simulink model "test_com_SensorFusion_SF_D4"  (R2019b)
settings: Solver=FixedStepDiscrete  StartTime=0  StopTime=stop  FixedStep=0.001  RelTol=1e-3
undefined symbols (not defined in the file or in its folder): BxTM, ByTM, CxTM, CyTM, g, gamma_stat_front, gamma_stat_rear, gearbox_ratio, l_F, l_R, m_sprung, m_unsprung_quarter, mag_calib_front_center, mag_calib_front_compmatrix, mag_calib_rear_center, mag_calib_rear_compmatrix, should_be_in_theSensorFusion, switch_VelYcalculation_pSF, testStart_VelX_pSF, testVelY_pSF, tire_r_dyn, track_angle_front, track_width_front, track_width_rear, v2o_x, wheel_kinematics_breakpoints, wheel_kinematics_FL_data, wheel_kinematics_FR_data, wheelbase, x9DFrontX, x9DFrontY, x9DRearX, x9DRearY
libraries: SignalProcessingSensorFusionLib x30, simulink x6
(part 2 of 9)

== system test_com_SensorFusion_SF_D4/0213_PlausibiltyCheck1/9DRear_Plausibility ==
  In : Inport  OutDataTypeStr=Bus: control_9D
  Bus Creator : BusCreator  Inputs=16  OutDataTypeStr=Bus: control_9D
  Bus Selector : BusSelector  OutputSignals=AccX,AccX_Sq,AccY,AccY_Sq,AccZ,AccZ_Sq,RollRate,RollRate_Sq,PitchRate,PitchRate_Sq,YawRate,YawRate_Sq,MagX,MagY,MagZ,Temperature
  Plausibility_Test_AccX : SignalProcessingSensorFusionLib/Plausibility_AllTests  alpha=0.3  checkGradient=off  deviation=0  threshold=0  alpha2=0  increasingPercentage=0  signalBounds=1e-8  stepDelay=25  upperBound=50  lowerBound=-50  useAlternativeValue=off  useManualAlternativeValue=off  manualAlternativeValue=0
  Plausibility_Test_AccY : SignalProcessingSensorFusionLib/Plausibility_AllTests  alpha=0.3  checkGradient=off  deviation=0  threshold=0  alpha2=0  increasingPercentage=0  signalBounds=1e-8  stepDelay=25  upperBound=50  lowerBound=-50  useAlternativeValue=off  useManualAlternativeValue=off  manualAlternativeValue=0
  Plausibility_Test_AccZ : SignalProcessingSensorFusionLib/Plausibility_AllTests  alpha=0.3  checkGradient=off  deviation=0  threshold=0  alpha2=0  increasingPercentage=0  signalBounds=1e-8  stepDelay=25  upperBound=50  lowerBound=-50  useAlternativeValue=off  useManualAlternativeValue=off  manualAlternativeValue=0
  Plausibility_Test_PitchRate : SignalProcessingSensorFusionLib/Plausibility_AllTests  alpha=0.3  checkGradient=off  deviation=0  threshold=0  alpha2=0  increasingPercentage=0  signalBounds=1e-8  stepDelay=25  upperBound=1.5  lowerBound=-1.5  useAlternativeValue=off  useManualAlternativeValue=off  manualAlternativeValue=0
  Plausibility_Test_RollRate : SignalProcessingSensorFusionLib/Plausibility_AllTests  alpha=0.3  checkGradient=off  deviation=0  threshold=0  alpha2=0  increasingPercentage=0  signalBounds=1e-8  stepDelay=25  upperBound=1.5  lowerBound=-1.5  useAlternativeValue=off  useManualAlternativeValue=off  manualAlternativeValue=0
  Plausibility_Test_YawRate : SignalProcessingSensorFusionLib/Plausibility_AllTests  alpha=0.3  checkGradient=off  deviation=0  threshold=0  alpha2=0  increasingPercentage=0  signalBounds=1e-8  stepDelay=25  upperBound=4  lowerBound=-4  useAlternativeValue=off  useManualAlternativeValue=off  manualAlternativeValue=0
  Scope : Scope  NumInputPorts=2
  Out : Outport  VectorParamsAs1DForOutWhenUnconnected=off
  wires:
  Plausibility_Test_AccY/1 -> Bus Creator/2  "AccY"
  Bus Selector/2 -> Plausibility_Test_AccX/2  "<AccX_Sq>"
  Bus Selector/4 -> Plausibility_Test_AccY/2  "<AccY_Sq>"
  Bus Selector/3 -> Plausibility_Test_AccY/1  "<AccY>"
  In/1 -> Bus Selector/1
  Plausibility_Test_AccX/1 -> Bus Creator/1  "AccX"
  Bus Selector/1 -> Plausibility_Test_AccX/1  "<AccX>"
  Bus Selector/6 -> Plausibility_Test_AccZ/2  "<AccZ_Sq>"
  Plausibility_Test_AccZ/1 -> Scope/1, Bus Creator/3  "AccZ"
  Bus Selector/5 -> Plausibility_Test_AccZ/1  "<AccZ>"
  Bus Selector/8 -> Plausibility_Test_RollRate/2  "<RollRate_Sq>"
  Bus Selector/7 -> Plausibility_Test_RollRate/1  "<RollRate>"
  Plausibility_Test_RollRate/1 -> Bus Creator/4  "RollRate"
  Bus Creator/1 -> Out/1
  Bus Selector/10 -> Plausibility_Test_PitchRate/2  "<PitchRate_Sq>"
  Plausibility_Test_PitchRate/1 -> Bus Creator/5  "PitchRate"
  Bus Selector/12 -> Plausibility_Test_YawRate/2  "<YawRate_Sq>"
  Plausibility_Test_YawRate/1 -> Bus Creator/6  "YawRate"
  Bus Selector/9 -> Plausibility_Test_PitchRate/1  "<PitchRate>"
  Bus Selector/11 -> Plausibility_Test_YawRate/1  "<YawRate>"
  Bus Selector/13 -> Bus Creator/7  "<MagX>"
  Bus Selector/14 -> Bus Creator/8  "<MagY>"
  Bus Selector/15 -> Bus Creator/9  "<MagZ>"
  Bus Selector/16 -> Bus Creator/10  "<Temperature>"
  Plausibility_Test_PitchRate/2 -> Bus Creator/15  "PitchRate_Sq"
  Plausibility_Test_AccZ/2 -> Scope/2, Bus Creator/13  "AccZ_Sq"
  Plausibility_Test_YawRate/2 -> Bus Creator/16  "YawRate_Sq"
  Plausibility_Test_AccX/2 -> Bus Creator/11  "AccX_Sq"
  Plausibility_Test_RollRate/2 -> Bus Creator/14  "RollRate_Sq"
  Plausibility_Test_AccY/2 -> Bus Creator/12  "AccY_Sq"

== system test_com_SensorFusion_SF_D4/0213_PlausibiltyCheck1/DriverRequest_Plausibility ==
  In : Inport  OutDataTypeStr=Bus: control_DriverRequest
  Bus Creator : BusCreator  Inputs=11  OutDataTypeStr=Bus: control_DriverRequest
      settings: InheritFromInputs=off
  Bus Selector : BusSelector  OutputSignals=Pedal_BrakeMech_Value,Pedal_BrakeRecu_Value,SteeringwheelAngle,Pedal_Accel_Value,Pedal_TorqueValid_flag,Pedal_BrakeHard_flag,Pedal_BrakeMech_flag,SteeringValid_flag,Pedal_BrakeValid_flag,SteeringwheelAngle_Sq,Pedal_Accel_Value_Sq
  Data Type Conrsion{1..3,22} (4 alike) : DataTypeConversion  OutDataTypeStr=single
  Data Type Conrsion{4..7} (4 alike) : DataTypeConversion  OutDataTypeStr=uint8
  Plausibility_Test_SteeringwheelAngle : SignalProcessingSensorFusionLib/Plausibility_AllTests  alpha=0.3  checkGradient=off  deviation=0  threshold=0  alpha2=0  increasingPercentage=0  signalBounds=1e-10  stepDelay=40  upperBound=115  lowerBound=-115  useAlternativeValue=off  useManualAlternativeValue=off  manualAlternativeValue=0
  Plausibility_Test_SteeringwheelAngle3 : SignalProcessingSensorFusionLib/Plausibility_AllTests  alpha=0.3  checkGradient=off  deviation=0  threshold=0  alpha2=0  increasingPercentage=0  signalBounds=1e-10  stepDelay=40  upperBound=1  lowerBound=0  useAlternativeValue=off  useManualAlternativeValue=off  manualAlternativeValue=0
  Out : Outport  VectorParamsAs1DForOutWhenUnconnected=off
  wires:
  In/1 -> Bus Selector/1
  Bus Creator/1 -> Out/1
  Bus Selector/1 -> Data Type Conrsion22/1  "<Pedal_BrakeMech_Value>"
  Bus Selector/2 -> Data Type Conrsion1/1  "<Pedal_BrakeRecu_Value>"
  Bus Selector/3 -> Plausibility_Test_SteeringwheelAngle/1  "<SteeringwheelAngle>"
  Plausibility_Test_SteeringwheelAngle/1 -> Data Type Conrsion2/1  "SteeringwheelAngle"
  Bus Selector/4 -> Plausibility_Test_SteeringwheelAngle3/1  "<Pedal_Accel_Value>"
  Bus Selector/5 -> Bus Creator/5  "<Pedal_TorqueValid_flag>"
  Bus Selector/6 -> Bus Creator/6  "<Pedal_BrakeHard_flag>"
  Bus Selector/7 -> Bus Creator/7  "<Pedal_BrakeMech_flag>"
  Bus Selector/8 -> Bus Creator/8  "<SteeringValid_flag>"
  Bus Selector/9 -> Bus Creator/9  "<Pedal_BrakeValid_flag>"
  Plausibility_Test_SteeringwheelAngle/2 -> Data Type Conrsion4/1  "SteeringwheelAngle_Sq"
  Plausibility_Test_SteeringwheelAngle3/1 -> Data Type Conrsion3/1
  Bus Selector/10 -> Data Type Conrsion6/1  "<SteeringwheelAngle_Sq>"
  Data Type Conrsion22/1 -> Bus Creator/1
  Data Type Conrsion1/1 -> Bus Creator/2
  Data Type Conrsion2/1 -> Bus Creator/3
  Data Type Conrsion3/1 -> Bus Creator/4
  Data Type Conrsion4/1 -> Bus Creator/10
  Bus Selector/11 -> Data Type Conrsion7/1  "<Pedal_Accel_Value_Sq>"
  Plausibility_Test_SteeringwheelAngle3/2 -> Data Type Conrsion5/1
  Data Type Conrsion5/1 -> Bus Creator/11
  Data Type Conrsion6/1 -> Plausibility_Test_SteeringwheelAngle/2
  Data Type Conrsion7/1 -> Plausibility_Test_SteeringwheelAngle3/2

== system test_com_SensorFusion_SF_D4/0213_PlausibiltyCheck1/Suspension_Plausibility ==
  In : Inport  OutDataTypeStr=Bus: control_Suspension
  Bus Creator : BusCreator  Inputs=8  OutDataTypeStr=Bus: control_Suspension
  Bus Selector : BusSelector  OutputSignals=RockerAngle_FL,RockerAngle_FL_Sq,RockerAngle_FR,RockerAngle_FR_Sq,RockerAngle_RL,RockerAngle_RL_Sq,RockerAngle_RR,RockerAngle_RR_Sq
  Data Type Conrsion{1..3,22} (4 alike) : DataTypeConversion  OutDataTypeStr=single
  Plausibility_Test_RockerAngle_FL : SignalProcessingSensorFusionLib/Plausibility_AllTests  alpha=0  checkGradient=off  deviation=0  threshold=0  alpha2=0  increasingPercentage=0  signalBounds=1e-10  stepDelay=38  upperBound=30  lowerBound=-30  useAlternativeValue=off  useManualAlternativeValue=off  manualAlternativeValue=0
  Plausibility_Test_RockerAngle_FR : SignalProcessingSensorFusionLib/Plausibility_AllTests  alpha=0  checkGradient=off  deviation=0  threshold=0  alpha2=0  increasingPercentage=0  signalBounds=1e-10  stepDelay=38  upperBound=30  lowerBound=-30  useAlternativeValue=off  useManualAlternativeValue=off  manualAlternativeValue=0
  Plausibility_Test_RockerAngle_RL : SignalProcessingSensorFusionLib/Plausibility_AllTests  alpha=0  checkGradient=off  deviation=0  threshold=0  alpha2=0  increasingPercentage=0  signalBounds=1e-10  stepDelay=38  upperBound=30  lowerBound=-30  useAlternativeValue=off  useManualAlternativeValue=off  manualAlternativeValue=0
  Plausibility_Test_RockerAngle_RR : SignalProcessingSensorFusionLib/Plausibility_AllTests  alpha=0  checkGradient=off  deviation=0  threshold=0  alpha2=0  increasingPercentage=0  signalBounds=1e-10  stepDelay=38  upperBound=30  lowerBound=-30  useAlternativeValue=off  useManualAlternativeValue=off  manualAlternativeValue=0
  Out : Outport  VectorParamsAs1DForOutWhenUnconnected=off
  wires:
  Plausibility_Test_RockerAngle_FL/2 -> Bus Creator/5  "RockerAngle_FL_Sq"
  Plausibility_Test_RockerAngle_FR/2 -> Bus Creator/6  "RockerAngle_FR_Sq"
  Plausibility_Test_RockerAngle_RL/2 -> Bus Creator/7  "RockerAngle_RL_Sq"
  Bus Selector/6 -> Plausibility_Test_RockerAngle_RL/2  "<RockerAngle_RL_Sq>"
  Bus Selector/5 -> Plausibility_Test_RockerAngle_RL/1  "<RockerAngle_RL>"
  Bus Selector/4 -> Plausibility_Test_RockerAngle_FR/2  "<RockerAngle_FR_Sq>"
  Bus Selector/3 -> Plausibility_Test_RockerAngle_FR/1  "<RockerAngle_FR>"
  Bus Selector/2 -> Plausibility_Test_RockerAngle_FL/2  "<RockerAngle_FL_Sq>"
  Bus Selector/1 -> Plausibility_Test_RockerAngle_FL/1  "<RockerAngle_FL>"
  Bus Creator/1 -> Out/1
  Plausibility_Test_RockerAngle_RL/1 -> Data Type Conrsion2/1
  Plausibility_Test_RockerAngle_FL/1 -> Data Type Conrsion22/1
  In/1 -> Bus Selector/1
  Plausibility_Test_RockerAngle_FR/1 -> Data Type Conrsion1/1
  Bus Selector/7 -> Plausibility_Test_RockerAngle_RR/1  "<RockerAngle_RR>"
  Plausibility_Test_RockerAngle_RR/2 -> Bus Creator/8  "RockerAngle_RR_Sq"
  Plausibility_Test_RockerAngle_RR/1 -> Data Type Conrsion3/1
  Bus Selector/8 -> Plausibility_Test_RockerAngle_RR/2  "<RockerAngle_RR_Sq>"
  Data Type Conrsion22/1 -> Bus Creator/1  "RockerAngle_FL"
  Data Type Conrsion1/1 -> Bus Creator/2  "RockerAngle_FR"
  Data Type Conrsion2/1 -> Bus Creator/3  "RockerAngle_RL"
  Data Type Conrsion3/1 -> Bus Creator/4  "RockerAngle_RR"

== system test_com_SensorFusion_SF_D4/0213_PlausibiltyCheck1/Suspension_Plausibility1 ==
  In : Inport  OutDataTypeStr=Bus: control_Electric
  Bus Creator : BusCreator  Inputs=12  OutDataTypeStr=Bus: control_Electric
  Bus Selector : BusSelector  OutputSignals=BatSOC,BatVoltage,BatPower,BatCurrent,AvgCellVoltage,MaxCellVoltage,MinCellVoltage,IVTEnergy,MinCellTemp,IVT_VoltageCurrent_Sq,IVT_Energy_Sq,HVM_BMS_Sq
  Data Type Conrsion22 : DataTypeConversion  OutDataTypeStr=single
  Plausibility_Test_RockerAngle_RL : SignalProcessingSensorFusionLib/Plausibility_AllTests  alpha=0  checkGradient=off  deviation=0  threshold=0  alpha2=0  increasingPercentage=0  signalBounds=1e-10  stepDelay=40  upperBound=120000  lowerBound=-120000  useAlternativeValue=off  useManualAlternativeValue=off  manualAlternativeValue=0
  Out : Outport  VectorParamsAs1DForOutWhenUnconnected=off
  wires:
  Bus Selector/8 -> Plausibility_Test_RockerAngle_RL/1  "<IVTEnergy>"
  Bus Selector/7 -> Bus Creator/7  "<MinCellVoltage>"
  In/1 -> Bus Selector/1
  Bus Creator/1 -> Out/1
  Bus Selector/1 -> Bus Creator/1  "<BatSOC>"
  Bus Selector/2 -> Bus Creator/2  "<BatVoltage>"
  Bus Selector/3 -> Bus Creator/3  "<BatPower>"
  Bus Selector/4 -> Bus Creator/4  "<BatCurrent>"
  Bus Selector/5 -> Bus Creator/5  "<AvgCellVoltage>"
  Bus Selector/6 -> Bus Creator/6  "<MaxCellVoltage>"
  Bus Selector/9 -> Bus Creator/9  "<MinCellTemp>"
  Bus Selector/10 -> Bus Creator/10  "<IVT_VoltageCurrent_Sq>"
  Bus Selector/11 -> Plausibility_Test_RockerAngle_RL/2  "<IVT_Energy_Sq>"
  Bus Selector/12 -> Bus Creator/12  "<HVM_BMS_Sq>"
  Plausibility_Test_RockerAngle_RL/2 -> Bus Creator/11  "AccZ_Sq"
  Plausibility_Test_RockerAngle_RL/1 -> Data Type Conrsion22/1  "VelZ"
  Data Type Conrsion22/1 -> Bus Creator/8

== system test_com_SensorFusion_SF_D4/0213_PlausibiltyCheck1/motorSpeed_Plausibility ==
  In : Inport
  Constant{,1..3} (4 alike) : Constant  Value=uint8(0)
  Data Type Conrsion22 : DataTypeConversion  OutDataTypeStr=single
  Demux : Demux
  Mux : Mux
  Mux1 : Mux
  Plausibility_Test_AccX : SignalProcessingSensorFusionLib/Plausibility_AllTests  alpha=0  checkGradient=off  deviation=0  threshold=0  alpha2=0  increasingPercentage=0  signalBounds=1e-10  stepDelay=40  upperBound=20000  lowerBound=-10000  useAlternativeValue=off  useManualAlternativeValue=off  manualAlternativeValue=0
  Plausibility_Test_AccY : SignalProcessingSensorFusionLib/Plausibility_AllTests  alpha=0  checkGradient=off  deviation=0  threshold=0  alpha2=0  increasingPercentage=0  signalBounds=1e-10  stepDelay=40  upperBound=20000  lowerBound=-10000  useAlternativeValue=off  useManualAlternativeValue=off  manualAlternativeValue=0
  Plausibility_Test_AccZ : SignalProcessingSensorFusionLib/Plausibility_AllTests  alpha=0  checkGradient=off  deviation=0  threshold=0  alpha2=0  increasingPercentage=0  signalBounds=1e-10  stepDelay=40  upperBound=20000  lowerBound=-10000  useAlternativeValue=off  useManualAlternativeValue=off  manualAlternativeValue=0
  Plausibility_Test_AccZ1 : SignalProcessingSensorFusionLib/Plausibility_AllTests  alpha=0  checkGradient=off  deviation=0  threshold=0  alpha2=0  increasingPercentage=0  signalBounds=1e-10  stepDelay=40  upperBound=20000  lowerBound=-10000  useAlternativeValue=off  useManualAlternativeValue=off  manualAlternativeValue=0
  WheelSpeed : Outport  VectorParamsAs1DForOutWhenUnconnected=off
  WheelSpeed_Sq : Outport  Port=2  VectorParamsAs1DForOutWhenUnconnected=off
  wires:
  Plausibility_Test_AccX/2 -> Mux1/1  "AccX_Sq"
  Plausibility_Test_AccZ1/2 -> Mux1/4
  Mux1/1 -> WheelSpeed_Sq/1
  Mux/1 -> Data Type Conrsion22/1
  Plausibility_Test_AccZ1/1 -> Mux/4
  Constant3/1 -> Plausibility_Test_AccZ1/2
  Constant2/1 -> Plausibility_Test_AccZ/2
  Constant1/1 -> Plausibility_Test_AccY/2
  Constant/1 -> Plausibility_Test_AccX/2
  Demux/4 -> Plausibility_Test_AccZ1/1
  Plausibility_Test_AccY/2 -> Mux1/2  "AccY_Sq"
  Plausibility_Test_AccZ/2 -> Mux1/3  "AccZ_Sq"
  Demux/3 -> Plausibility_Test_AccZ/1
  Demux/2 -> Plausibility_Test_AccY/1
  Demux/1 -> Plausibility_Test_AccX/1
  Plausibility_Test_AccZ/1 -> Mux/3  "VelZ"
  Plausibility_Test_AccX/1 -> Mux/1  "VelX"
  In/1 -> Demux/1  "wheelSpeed"
  Plausibility_Test_AccY/1 -> Mux/2  "VelY"
  Data Type Conrsion22/1 -> WheelSpeed/1

== system test_com_SensorFusion_SF_D4/0213_PlausibiltyCheck1/v2oVelocity_Plausibility ==
  In : Inport  OutDataTypeStr=Bus: control_Velocity
  Bus Creator : BusCreator  Inputs=7  OutDataTypeStr=Bus: control_Velocity
  Bus Creator1 : BusCreator  Inputs=2
  Bus Creator2 : BusCreator  Inputs=2
  Bus Selector : BusSelector  OutputSignals=SlipAngle,SlipAngle_Sq,VelY,VelY_Sq,VelX,VelX_Sq,valueIsNew
  Bus Selector1 : BusSelector  OutputSignals=VelY,VelX,VelY_Sq,VelX_Sq
  Data Type Conrsion1 : DataTypeConversion  OutDataTypeStr=single
  Data Type Conrsion2 : DataTypeConversion  OutDataTypeStr=single
  Data Type Conrsion22 : DataTypeConversion  OutDataTypeStr=single
  Plausibility_Test_SlipAngle : SignalProcessingSensorFusionLib/Plausibility_AllTests  alpha=0  checkGradient=off  deviation=0  threshold=0  alpha2=0  increasingPercentage=0  signalBounds=1e-8  stepDelay=35  upperBound=90  lowerBound=-90  useAlternativeValue=off  useManualAlternativeValue=off  manualAlternativeValue=0
  Plausibility_Test_VelX : SignalProcessingSensorFusionLib/Plausibility_AllTests  alpha=0  checkGradient=off  deviation=0  threshold=0  alpha2=0  increasingPercentage=0  signalBounds=1e-8  stepDelay=35  upperBound=35  lowerBound=-3  useAlternativeValue=off  useManualAlternativeValue=off  manualAlternativeValue=0
  Plausibility_Test_VelY : SignalProcessingSensorFusionLib/Plausibility_AllTests  alpha=0  checkGradient=off  deviation=0  threshold=0  alpha2=0  increasingPercentage=0  signalBounds=1e-8  stepDelay=35  upperBound=50  lowerBound=-50  useAlternativeValue=off  useManualAlternativeValue=off  manualAlternativeValue=0
  Scope : Scope  NumInputPorts=2
  Out : Outport  VectorParamsAs1DForOutWhenUnconnected=off
  wires:
  Plausibility_Test_VelY/1 -> Data Type Conrsion22/1  "VelY"
  In/1 -> Bus Selector/1
  Plausibility_Test_SlipAngle/1 -> Data Type Conrsion1/1  "SlipAngle"
  Plausibility_Test_VelX/1 -> Data Type Conrsion2/1  "VelX"
  Bus Creator/1 -> Bus Selector1/1, Out/1
  Bus Selector/1 -> Plausibility_Test_SlipAngle/1  "<SlipAngle>"
  Bus Selector/2 -> Plausibility_Test_SlipAngle/2  "<SlipAngle_Sq>"
  Bus Selector/3 -> Plausibility_Test_VelY/1  "<VelY>"
  Bus Selector/4 -> Plausibility_Test_VelY/2  "<VelY_Sq>"
  Bus Selector/5 -> Plausibility_Test_VelX/1  "<VelX>"
  Bus Selector/6 -> Plausibility_Test_VelX/2  "<VelX_Sq>"
  Bus Selector/7 -> Bus Creator/7  "<valueIsNew>"
  Plausibility_Test_VelX/2 -> Bus Creator/6  "VelX_Sq"
  Plausibility_Test_VelY/2 -> Bus Creator/5  "VelY_Sq"
  Plausibility_Test_SlipAngle/2 -> Bus Creator/4  "SlipAngle_Sq"
  Data Type Conrsion22/1 -> Bus Creator/2  "VelY"
  Data Type Conrsion1/1 -> Bus Creator/1  "SlipAngle"
  Data Type Conrsion2/1 -> Bus Creator/3  "VelX"
  Bus Selector1/1 -> Bus Creator1/1  "<VelY>"
  Bus Selector1/2 -> Bus Creator1/2  "<VelX>"
  Bus Selector1/3 -> Bus Creator2/1  "<VelY_Sq>"
  Bus Selector1/4 -> Bus Creator2/2  "<VelX_Sq>"
  Bus Creator2/1 -> Scope/2
  Bus Creator1/1 -> Scope/1

== system test_com_SensorFusion_SF_D4/0213_PlausibiltyCheck1/wheelSpeed_Plausibility ==
  In : Inport
  Constant{,1..3} (4 alike) : Constant  Value=uint8(0)
  Data Type Conrsion{1..3,22} (4 alike) : DataTypeConversion  OutDataTypeStr=single
  Demux : Demux
  Mux : Mux
  Mux1 : Mux
  Plausibility_Test_WheelSpeed_FL : SignalProcessingSensorFusionLib/Plausibility_AllTests  alpha=0  checkGradient=off  deviation=0  threshold=0  alpha2=0  increasingPercentage=0  signalBounds=1e-12  stepDelay=40  upperBound=100  lowerBound=-10  useAlternativeValue=off  useManualAlternativeValue=off  manualAlternativeValue=0
  Plausibility_Test_WheelSpeed_FR : SignalProcessingSensorFusionLib/Plausibility_AllTests  alpha=0  checkGradient=off  deviation=0  threshold=0  alpha2=0  increasingPercentage=0  signalBounds=1e-12  stepDelay=40  upperBound=100  lowerBound=-10  useAlternativeValue=off  useManualAlternativeValue=off  manualAlternativeValue=0
  Plausibility_Test_WheelSpeed_RL : SignalProcessingSensorFusionLib/Plausibility_AllTests  alpha=0  checkGradient=off  deviation=0  threshold=0  alpha2=0  increasingPercentage=0  signalBounds=1e-12  stepDelay=40  upperBound=100  lowerBound=-10  useAlternativeValue=off  useManualAlternativeValue=off  manualAlternativeValue=0
  Plausibility_Test_WheelSpeed_RR : SignalProcessingSensorFusionLib/Plausibility_AllTests  alpha=0  checkGradient=off  deviation=0  threshold=0  alpha2=0  increasingPercentage=0  signalBounds=1e-12  stepDelay=40  upperBound=100  lowerBound=-10  useAlternativeValue=off  useManualAlternativeValue=off  manualAlternativeValue=0
  WheelSpeed : Outport  VectorParamsAs1DForOutWhenUnconnected=off
  WheelSpeed_Sq : Outport  Port=2  VectorParamsAs1DForOutWhenUnconnected=off
  wires:
  Plausibility_Test_WheelSpeed_FR/1 -> Data Type Conrsion1/1  "VelY"
  In/1 -> Demux/1  "wheelSpeed"
  Plausibility_Test_WheelSpeed_FL/1 -> Data Type Conrsion22/1  "VelX"
  Plausibility_Test_WheelSpeed_RL/1 -> Data Type Conrsion2/1  "VelZ"
  Demux/1 -> Plausibility_Test_WheelSpeed_FL/1
  Demux/2 -> Plausibility_Test_WheelSpeed_FR/1
  Demux/3 -> Plausibility_Test_WheelSpeed_RL/1
  Plausibility_Test_WheelSpeed_RL/2 -> Mux1/3  "AccZ_Sq"
  Plausibility_Test_WheelSpeed_FR/2 -> Mux1/2  "AccY_Sq"
  Demux/4 -> Plausibility_Test_WheelSpeed_RR/1
  Constant/1 -> Plausibility_Test_WheelSpeed_FL/2
  Constant1/1 -> Plausibility_Test_WheelSpeed_FR/2
  Constant2/1 -> Plausibility_Test_WheelSpeed_RL/2
  Constant3/1 -> Plausibility_Test_WheelSpeed_RR/2
  Plausibility_Test_WheelSpeed_RR/1 -> Data Type Conrsion3/1
  Mux/1 -> WheelSpeed/1
  Mux1/1 -> WheelSpeed_Sq/1
  Plausibility_Test_WheelSpeed_RR/2 -> Mux1/4
  Plausibility_Test_WheelSpeed_FL/2 -> Mux1/1  "AccX_Sq"
  Data Type Conrsion22/1 -> Mux/1
  Data Type Conrsion1/1 -> Mux/2
  Data Type Conrsion2/1 -> Mux/3
  Data Type Conrsion3/1 -> Mux/4

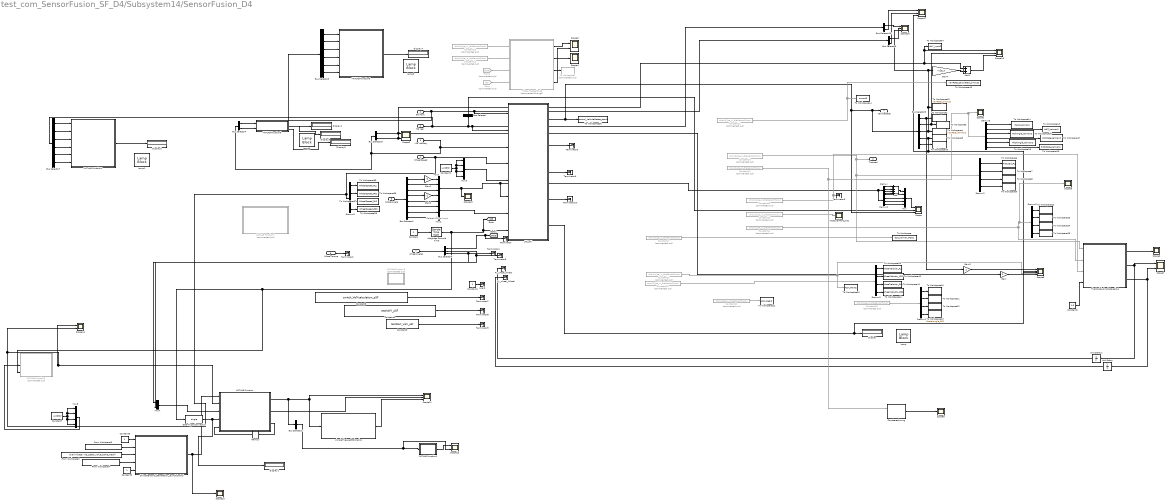
== system test_com_SensorFusion_SF_D4/Subsystem14/SensorFusion_D4 ==
  note: Deleted Driver Input
  9D front : Inport
  9D rear : Inport  Port=2
  v2o velocity : Inport  Port=3
  WheelSpeed : Inport  Port=4
  RockerAngle : Inport  Port=5
  WheelTorque : Inport  Port=6
  WheelAngle1 : Inport  Port=7
  Add : Sum  Inputs=++++
  Add1 : Sum
  Bus Selector : BusSelector  OutputSignals=AccX,AccY,AccZ,RollRate,PitchRate,YawRate  OutputAsBus=on
  Bus Selector1 : BusSelector  OutputSignals=RockerAngle_FL,RockerAngle_FR,RockerAngle_RL,RockerAngle_RR,RockerAngle_FL_Sq,RockerAngle_FR_Sq,RockerAngle_RL_Sq,RockerAngle_RR_Sq
  Bus Selector10 : BusSelector  OutputSignals=YawRate,AccX
  Bus Selector2 : BusSelector  OutputSignals=AccX
  Bus Selector3 : BusSelector  OutputSignals=VelX,VelY
  Bus Selector4 : BusSelector  OutputSignals=VelX_Sq,VelY_Sq
  Bus Selector5 : BusSelector  OutputSignals=VelX,VelY,YawRate,AccX,AccY
  Bus Selector6 : BusSelector  OutputSignals=WheelAngle_AVG,WheelAngle_FL,WheelAngle_FR
  Bus Selector7 : BusSelector  OutputSignals=AccX_Sq,AccY_Sq,AccZ_Sq,YawRate_Sq,PitchRate_Sq,RollRate_Sq
  Bus Selector8 : BusSelector  OutputSignals=AccX_Sq,AccY_Sq,AccZ_Sq,YawRate_Sq,PitchRate_Sq,RollRate_Sq
  Bus Selector9 : BusSelector  OutputSignals=YawRate,AccX
  Constant{,4..6} (4 alike) : Constant
  Constant1 : Constant  Value=uint8(0)
  Constant{10..22} (13 alike) : Constant  Commented=on  Value=should_be_in_theSensorFusion
  Constant2 : Constant  Value=1.6
  Constant3 : Constant  Value=testVelY_pSF
  Constant7 : Constant  Value=uint8(0)
  Constant8 : Constant  Value=switch_VelYcalculation_pSF
  Constant9 : Constant  Value=testStart_VelX_pSF
  Data Type Conversion : DataTypeConversion  OutDataTypeStr=single
  Demux{,1..2,4..5,8..9} (7 alike) : Demux
  Demux3 : Demux  Outputs=6
  Display{,1..6} (7 alike) : Display
  DriverDemand_Generation_LaunchControl : Subsystem
  From : From  Commented=on  GotoTag=dt
  From Workspace2 : FromWorkspace  VariableName=evalin('base','VD_pedal_value_brake_mech')  SampleTime=0
  From Workspace3 : FromWorkspace  VariableName=evalin('base','VD_pedal_value_brake_rec')  SampleTime=0
  From Workspace4 : FromWorkspace  VariableName=evalin('base','VD_pedal_value_torque')  SampleTime=0
  From1 : From  Commented=on  GotoTag=delta
  Fx_wheel_Wheel : Terminator
  Fy_wheel_Wheel : Terminator
  Gain : Gain  OutDataTypeStr=single
  Gain1 : Gain  Gain=-1
  Gain2 : Gain  Gain=-1
  Gain3 : Gain  OutDataTypeStr=single
  Gain4 : Gain  Gain=-v2o_x
  Lamp{,1..3} (4 alike) : LampBlock
  MATLAB Function : MATLAB Function  TreatAsAtomicUnit=on
  MATLAB Function1 : MATLAB Function  TreatAsAtomicUnit=on
  MATLAB Function2 : MATLAB Function  Commented=on  TreatAsAtomicUnit=on
  MATLAB Function3 : MATLAB Function  Commented=on  TreatAsAtomicUnit=on
  MATLAB Function4 : MATLAB Function  TreatAsAtomicUnit=on
  MATLAB Function5 : MATLAB Function  TreatAsAtomicUnit=on
  MATLAB Function6 : MATLAB Function  TreatAsAtomicUnit=on
  MATLAB Function7 : MATLAB Function  Commented=on  TreatAsAtomicUnit=on
  Memory : Memory
  Mux : Mux  Inputs=5
  Mux{1..3,5} (4 alike) : Mux
  Mux4 : Mux  Inputs=2
  SF_LaKl : MATLAB Function  TreatAsAtomicUnit=on
  Scope{,11,15..17} (5 alike) : Scope  NumInputPorts=3
  Scope{1..2,4,6,9..10,13} (7 alike) : Scope
  Scope{3,5,7,12,14} (5 alike) : Scope  NumInputPorts=2
  Scope8 : Scope  NumInputPorts=5
  SiDes Testgelände : MATLAB Function  Commented=through  TreatAsAtomicUnit=on
  Sturzberechnung : Subsystem
  Terminator{,1..10} (11 alike) : Terminator
  TireModel_simplePacejka1 : MATLAB Function  TreatAsAtomicUnit=on
  To Workspace : ToWorkspace  VariableName=e10_kalman_POS2  SaveFormat=Timeseries  SampleTime=-1
  To Workspace1 : ToWorkspace  Commented=on  VariableName=e10_easy_POS  SaveFormat=Timeseries  SampleTime=-1
  To Workspace10 : ToWorkspace  VariableName=RockerAngle_FL2  SaveFormat=Timeseries  SampleTime=-1
  To Workspace11 : ToWorkspace  VariableName=RockerAngle_FR2  SaveFormat=Timeseries  SampleTime=-1
  To Workspace12 : ToWorkspace  VariableName=RockerAngle_RL2  SaveFormat=Timeseries  SampleTime=-1
  To Workspace13 : ToWorkspace  VariableName=RockerAngle_RR2  SaveFormat=Timeseries  SampleTime=-1
  To Workspace14 : ToWorkspace  VariableName=PosZ_kalman2  SaveFormat=Timeseries  SampleTime=-1
  To Workspace15 : ToWorkspace  VariableName=VelZ_kalman2  SaveFormat=Timeseries  SampleTime=-1
  To Workspace16 : ToWorkspace  VariableName=RollAngle_kalman2  SaveFormat=Timeseries  SampleTime=-1
  To Workspace17 : ToWorkspace  VariableName=RollRate_kalman2  SaveFormat=Timeseries  SampleTime=-1
  To Workspace18 : ToWorkspace  VariableName=PitchAngle_kalman2  SaveFormat=Timeseries  SampleTime=-1
  To Workspace19 : ToWorkspace  VariableName=PitchRate_kalman2  SaveFormat=Timeseries  SampleTime=-1
  To Workspace2 : ToWorkspace  VariableName=VelX_kalman2  SaveFormat=Timeseries  SampleTime=-1
  To Workspace20 : ToWorkspace  VariableName=AccX_Front2  SaveFormat=Timeseries  SampleTime=-1
  To Workspace21 : ToWorkspace  VariableName=AccX_Rear2  SaveFormat=Timeseries  SampleTime=-1
  To Workspace22 : ToWorkspace  VariableName=TireSlipLong_FL2  SaveFormat=Timeseries  SampleTime=-1
  To Workspace23 : ToWorkspace  VariableName=TireSlipLong_FR2  SaveFormat=Timeseries  SampleTime=-1
  To Workspace24 : ToWorkspace  VariableName=TireSlipLong_RL2  SaveFormat=Timeseries  SampleTime=-1
  To Workspace25 : ToWorkspace  VariableName=TireSlipLong_RR2  SaveFormat=Timeseries  SampleTime=-1
  To Workspace26 : ToWorkspace  VariableName=control_VehicleStates_result  SaveFormat=Timeseries  SampleTime=-1
  To Workspace3 : ToWorkspace  VariableName=VelY_kalman2  SaveFormat=Timeseries  SampleTime=-1
  To Workspace34 : ToWorkspace  VariableName=VelY_input2  SaveFormat=Timeseries  SampleTime=-1
  To Workspace35 : ToWorkspace  VariableName=WheelSpeed_FL2  SaveFormat=Timeseries  SampleTime=-1
  To Workspace36 : ToWorkspace  VariableName=WheelSpeed_FR2  SaveFormat=Timeseries  SampleTime=-1
  To Workspace37 : ToWorkspace  VariableName=WheelSpeed_RL2  SaveFormat=Timeseries  SampleTime=-1
  To Workspace38 : ToWorkspace  VariableName=WheelSpeed_RR2  SaveFormat=Timeseries  SampleTime=-1
  To Workspace39 : ToWorkspace  VariableName=WheelVelocity_FL2  SaveFormat=Timeseries  SampleTime=-1
  To Workspace4 : ToWorkspace  VariableName=YawRate_kalman2  SaveFormat=Timeseries  SampleTime=-1
  To Workspace40 : ToWorkspace  VariableName=WheelVelocity_FR2  SaveFormat=Timeseries  SampleTime=-1
  To Workspace41 : ToWorkspace  VariableName=WheelVelocity_RL2  SaveFormat=Timeseries  SampleTime=-1
  To Workspace42 : ToWorkspace  VariableName=WheelVelocity_RR2  SaveFormat=Timeseries  SampleTime=-1
  To Workspace43 : ToWorkspace  VariableName=AccY_kalman2  SaveFormat=Timeseries  SampleTime=-1
  To Workspace44 : ToWorkspace  VariableName=simout2  SaveFormat=Timeseries  SampleTime=-1
  To Workspace45 : ToWorkspace  VariableName=YawRate_simout2  SaveFormat=Timeseries  SampleTime=-1
  To Workspace46 : ToWorkspace  VariableName=YawRate_Calculated_simout2  SaveFormat=Timeseries  SampleTime=-1
  To Workspace5 : ToWorkspace  VariableName=AccX_kalman2  SaveFormat=Timeseries  SampleTime=-1
  To Workspace6 : ToWorkspace  VariableName=TireLoad_FL2  SaveFormat=Timeseries  SampleTime=-1
  To Workspace7 : ToWorkspace  VariableName=TireLoad_FR2  SaveFormat=Timeseries  SampleTime=-1
  To Workspace8 : ToWorkspace  VariableName=TireLoad_RL2  SaveFormat=Timeseries  SampleTime=-1
  To Workspace9 : ToWorkspace  VariableName=TireLoad_RR2  SaveFormat=Timeseries  SampleTime=-1
  Unit Delay : UnitDelay  SampleTime=-1  HasFrameUpgradeWarning=on
  Unit Delay1 : UnitDelay  SampleTime=-1  HasFrameUpgradeWarning=on
  Weighted Sample Time : SampleTimeMath  TsampMathOp=Ts Only
  c_reib : Terminator
  measurement_bias : Scope
  simpleTireLoadEstimation : Subsystem
  VehicleState : Outport  VectorParamsAs1DForOutWhenUnconnected=off
  TireLoad : Outport  Port=2  VectorParamsAs1DForOutWhenUnconnected=off
  wires:
  Mux/1 -> Scope/1
  Demux1/4 -> Mux/5
  Demux1/3 -> Mux/4
  Demux1/2 -> Mux/3
  Demux1/1 -> Mux/2
  Add/1 -> Mux/1
  Demux/1 -> Add/1
  Demux/2 -> Add/2
  Demux/3 -> Add/3
  Demux/4 -> Add/4
  Bus Selector/1 -> Scope/2
  Gain2/1 -> Mux1/4
  Weighted Sample Time/1 -> MATLAB Function2/3(dt), Data Type Conversion/1, [dt], SF_LaKl/8(dt)
  Mux2/1 -> SF_LaKl/7(RockerAngle_Sq)
  Mux1/1 -> Scope10/1, Demux/1, Demux1/1, SF_LaKl/6(RockerAngle)
  Mux3/1 -> SF_LaKl/5(WheelSpeeds_Sq)
  Gain1/1 -> Mux1/1
  v2o velocity/1 -> SF_LaKl/3(v2o), Bus Selector4/1, Bus Selector3/1
  9D rear/1 -> Bus Selector7/1, Bus Selector10/1, SF_LaKl/2(x9DRear), Bus Selector/1
  Bus Selector1/5 -> Mux2/1  "<RockerAngle_FL_Sq>"
  Constant/1 -> Weighted Sample Time/1
  Constant1/1 -> Mux3/2, Mux3/1, Mux3/3, Mux3/4
  Constant10/1 -> TireModel_simplePacejka1/1(TireLoad), Demux2/1, TireLoad/1  "TireLoad"
  Bus Selector1/7 -> Mux2/3  "<RockerAngle_RL_Sq>"
  Bus Selector1/8 -> Mux2/4  "<RockerAngle_RR_Sq>"
  Bus Selector1/3 -> Mux1/3  "<RockerAngle_RL>"
  Bus Selector1/4 -> Gain2/1  "<RockerAngle_RR>"
  WheelTorque/1 -> Terminator1/1
  RockerAngle/1 -> Bus Selector1/1  "rockerAngle"
  Bus Selector1/1 -> Gain1/1  "<RockerAngle_FL>"
  Bus Selector1/2 -> Mux1/2  "<RockerAngle_FR>"
  Constant13/1 -> SiDes Testgelände/2(x)
  SF_LaKl/1(VehicleState) -> To Workspace26/1, Scope/3, Bus Selector5/1, VehicleState/1  "VehicleState"
  Bus Selector1/6 -> Mux2/2  "<RockerAngle_FR_Sq>"
  Constant17/1 -> To Workspace/1
  Constant16/1 -> measurement_bias/1
  Constant19/1 -> SiDes Testgelände/1(measurements_nb)
  SiDes Testgelände/3(easyPos_out) -> To Workspace1/1
  SiDes Testgelände/1(easyYawRate_out) -> Scope3/1
  SiDes Testgelände/2(easyYawAngle_out) -> Scope4/1
  From/1 -> SiDes Testgelände/4(dt)
  From1/1 -> SiDes Testgelände/3(delta)
  SiDes Testgelände/4(YawRateBySteer) -> Scope3/2
  Bus Selector3/1 -> Gain/1, Scope5/1  "<VelX>"
  Bus Selector3/2 -> Add1/1, Scope15/1, To Workspace34/1, Scope5/2  "<VelY>"
  Bus Selector6/2 -> Terminator5/1, Mux4/1  "<WheelAngle_FL>"
  Bus Selector6/3 -> Terminator4/1, Mux4/2  "<WheelAngle_FR>"
  WheelAngle1/1 -> Bus Selector6/1
  Bus Selector6/1 -> Terminator/1, [delta]  "<WheelAngle_AVG>"
  9D front/1 -> Bus Selector8/1, Bus Selector9/1, SF_LaKl/1(x9DFront)
  Bus Selector5/1 -> Gain3/1, To Workspace2/1  "<VelX>"
  Bus Selector5/2 -> Scope15/2, To Workspace3/1  "<VelY>"
  Bus Selector5/3 -> To Workspace45/1, Scope16/3, Gain4/1, To Workspace4/1  "<YawRate>"
  Bus Selector5/4 -> Scope17/3, Scope8/2, To Workspace5/1  "<AccX>"
  Demux2/4 -> To Workspace9/1
  Demux2/3 -> To Workspace8/1
  Demux2/2 -> To Workspace7/1
  Demux2/1 -> To Workspace6/1
  Constant18/1 -> Demux4/1
  Demux3/1 -> To Workspace14/1
  Demux3/2 -> To Workspace15/1
  Demux3/3 -> To Workspace16/1
  Demux3/4 -> To Workspace17/1
  Demux3/5 -> To Workspace18/1
  Demux3/6 -> To Workspace19/1
  Demux4/1 -> To Workspace10/1
  Demux4/2 -> To Workspace11/1
  Demux4/3 -> To Workspace12/1
  Demux4/4 -> To Workspace13/1
  Demux5/4 -> To Workspace25/1
  Demux5/3 -> To Workspace24/1
  Demux5/2 -> To Workspace23/1
  Demux5/1 -> To Workspace22/1
  Constant14/1 -> TireModel_simplePacejka1/2(TireSlipLong), Scope9/1, Demux5/1
  Demux8/1 -> To Workspace35/1
  Demux8/2 -> To Workspace36/1
  Demux8/3 -> To Workspace37/1
  Demux8/4 -> To Workspace38/1
  Demux9/4 -> To Workspace42/1
  Demux9/3 -> To Workspace41/1
  Demux9/2 -> To Workspace40/1
  Constant20/1 -> Demux9/1
  Demux9/1 -> To Workspace39/1
  Bus Selector5/5 -> To Workspace43/1  "<AccY>"
  Constant15/1 -> TireModel_simplePacejka1/3(TireSlipAngle), Terminator3/1
  Constant12/1 -> To Workspace46/1, To Workspace44/1
  TireModel_simplePacejka1/1(TireLoadEff) -> Scope2/1
  TireModel_simplePacejka1/2(TireForceLong) -> Unit Delay1/1, Scope7/1
  Constant2/1 -> TireModel_simplePacejka1/4(mux_nominal)
  Constant4/1 -> c_reib/1
  TireModel_simplePacejka1/3(TireForceLat) -> Scope7/2, Unit Delay/1
  Constant21/1 -> To Workspace20/1, Scope8/4
  Constant22/1 -> To Workspace21/1
  Unit Delay/1 -> Fy_wheel_Wheel/1
  Unit Delay1/1 -> Fx_wheel_Wheel/1
  Constant11/1 -> Sturzberechnung/1(Orientation), Demux3/1, Scope1/1
  Sturzberechnung/1(CamberAngle) -> Scope6/1
  SF_LaKl/5(kalman_running) -> Scope8/3, Display/1
  Gain/1 -> Scope8/5  "VelX_sensor"
  Gain3/1 -> Scope8/1  "VelX_kalman"
  simpleTireLoadEstimation/1(TireLoad) -> Scope11/3
  Memory/1 -> MATLAB Function/5(WheelVelocity_old)
  MATLAB Function/2(TireSlipLong) -> Scope11/2
  MATLAB Function/3(WheelVelocity) -> Memory/1
  Mux4/1 -> MATLAB Function/3(WheelAngle)
  DriverDemand_Generation_LaunchControl/1(DriverDemand) -> Scope13/1, MATLAB Function/1(DriverDemand)
  Constant5/1 -> DriverDemand_Generation_LaunchControl/5(Driver)
  Constant6/1 -> DriverDemand_Generation_LaunchControl/1(DrivingMode)
  From Workspace2/1 -> DriverDemand_Generation_LaunchControl/3(Pedal_BrakeMechValue)  "MechBremspedal"
  From Workspace3/1 -> DriverDemand_Generation_LaunchControl/2(PedalBrakeRecuValue)  "RekuBremspedal"
  From Workspace4/1 -> DriverDemand_Generation_LaunchControl/4(PedalAccelValue)  "ms_ad_pedal_value_torque"
  Data Type Conversion/1 -> Display1/1, MATLAB Function/4(dt)
  MATLAB Function/1(VehicleState) -> Bus Selector2/1, simpleTireLoadEstimation/1(VehicleState), Scope11/1
  Bus Selector2/1 -> Scope12/2, MATLAB Function1/1(u)  "<AccX>"
  MATLAB Function1/1(y) -> Scope12/1
  WheelSpeed/1 -> SF_LaKl/4(WheelSpeeds), MATLAB Function/2(WheelSpeeds), Scope14/1, Scope14/2, Demux8/1
  Constant7/1 -> Mux5/2, Mux5/1, Mux5/3, Mux5/4
  Mux5/1 -> MATLAB Function2/2(WheelSpeeds_Sq)
  Bus Selector4/1 -> MATLAB Function5/1(VelX_Sq)  "<VelX_Sq>"
  Bus Selector4/2 -> MATLAB Function5/2(VelY_Sq)  "<VelY_Sq>"
  MATLAB Function5/1(VD_diag_v2o) -> Display2/1  "VD_diag_9Drear"
  Bus Selector7/1 -> MATLAB Function4/1(AccX_Sq)  "<AccX_Sq>"
  Bus Selector7/2 -> MATLAB Function4/2(AccY_Sq)  "<AccY_Sq>"
  Bus Selector7/3 -> MATLAB Function4/3(AccZ_Sq)  "<AccZ_Sq>"
  Bus Selector7/4 -> MATLAB Function4/4(YawRate_Sq)  "<YawRate_Sq>"
  Bus Selector7/5 -> MATLAB Function4/5(PitchRate_Sq)  "<PitchRate_Sq>"
  Bus Selector7/6 -> MATLAB Function4/6(RollRate_Sq)  "<RollRate_Sq>"
  MATLAB Function4/1(VD_diag_9Drear) -> Display3/1  "VD_diag_9Drear"
  Bus Selector8/1 -> MATLAB Function6/1(AccX_Sq)  "<AccX_Sq>"
  Bus Selector8/2 -> MATLAB Function6/2(AccY_Sq)  "<AccY_Sq>"
  Bus Selector8/6 -> MATLAB Function6/6(RollRate_Sq)  "<RollRate_Sq>"
  Bus Selector8/5 -> MATLAB Function6/5(PitchRate_Sq)  "<PitchRate_Sq>"
  Bus Selector8/4 -> MATLAB Function6/4(YawRate_Sq)  "<YawRate_Sq>"
  Bus Selector8/3 -> MATLAB Function6/3(AccZ_Sq)  "<AccZ_Sq>"
  MATLAB Function6/1(VD_diag_9Dfront) -> Display4/1  "VD"
  MATLAB Function5/2(bad_Sq_counter) -> Display5/1  "bad_SqCounter"
  MATLAB Function5/3(timestep_counter) -> Display6/1  "timestep_counter"
  Constant8/1 -> Terminator7/1
  Constant3/1 -> Terminator8/1
  Gain4/1 -> Add1/2
  Add1/1 -> Scope15/3
  Bus Selector10/1 -> Scope16/1  "<YawRate>"
  Bus Selector9/1 -> Scope16/2  "<YawRate>"
  Bus Selector10/2 -> Scope17/1  "<AccX>"
  Bus Selector9/2 -> Scope17/2  "<AccX>"
  Constant9/1 -> Terminator9/1
  SF_LaKl/2(used_bias) -> Terminator2/1  "bias_used_kalman_SiDe"
  SF_LaKl/3(used_measurements) -> Terminator6/1  "measurements_used_kalman_SiDe"
  SF_LaKl/4(bias_measurement_running) -> Terminator10/1  "bias_running_SiDe"
